simulink model "pneumatics"  (R2025a)
settings: Solver=FixedStepAuto  StartTime=0.0  StopTime=10  FixedStep=0.05  RelTol=1e-3
model workspace (MAT data in the model file):
  BP_MAX_SERVICE_REDUCTION = Simulink.Parameter
  BP_MAX_SERVICE_REDUCTION.Value = 25
  BP_MAX_SERVICE_REDUCTION.Complexity = 'real'
  BP_MAX_SERVICE_REDUCTION.Dimensions = [1 1]
  BP_MAX_SERVICE_REDUCTION.DataType = 'auto'
  BP_MAX_SERVICE_REDUCTION.DocUnits = 'psig'
  BP_NOMINAL_PRESSURE = Simulink.Parameter
  BP_NOMINAL_PRESSURE.Value = 90
  BP_NOMINAL_PRESSURE.Complexity = 'real'
  BP_NOMINAL_PRESSURE.Dimensions = [1 1]
  BP_NOMINAL_PRESSURE.DataType = 'auto'
  BP_NOMINAL_PRESSURE.DocUnits = 'psig'
  MAIN_RES_NOMINAL_PRESSURE = Simulink.Parameter
  MAIN_RES_NOMINAL_PRESSURE.Value = 164.69
  MAIN_RES_NOMINAL_PRESSURE.Complexity = 'real'
  MAIN_RES_NOMINAL_PRESSURE.Dimensions = [1 1]
  MAIN_RES_NOMINAL_PRESSURE.DataType = 'auto'
  MAIN_RES_NOMINAL_PRESSURE.DocUnits = 'psig'
  RESERVOIR_TEMPERATURE = Simulink.Parameter
  RESERVOIR_TEMPERATURE.Value = 75
  RESERVOIR_TEMPERATURE.Complexity = 'real'
  RESERVOIR_TEMPERATURE.Dimensions = [1 1]
  RESERVOIR_TEMPERATURE.DataType = 'auto'
  RESERVOIR_TEMPERATURE.DocUnits = '°F'
  RESERVOIR_VOLUME = Simulink.Parameter
  RESERVOIR_VOLUME.Value = 10
  RESERVOIR_VOLUME.Complexity = 'real'
  RESERVOIR_VOLUME.Dimensions = [1 1]
  RESERVOIR_VOLUME.DataType = 'auto'
  RESERVOIR_VOLUME.DocUnits = 'gal'
  TRANSDUCER_ADC_OUTPUT_RANGE = Simulink.Parameter
  TRANSDUCER_ADC_OUTPUT_RANGE.Value = 1019
  TRANSDUCER_ADC_OUTPUT_RANGE.Complexity = 'real'
  TRANSDUCER_ADC_OUTPUT_RANGE.Dimensions = [1 1]
  TRANSDUCER_ADC_OUTPUT_RANGE.DataType = 'auto'
  TRANSDUCER_ADC_OUTPUT_RANGE.DocUnits = 'bit'
  TRANSDUCER_OUTPUT_HIGH = Simulink.Parameter
  TRANSDUCER_OUTPUT_HIGH.Value = 4.5
  TRANSDUCER_OUTPUT_HIGH.Complexity = 'real'
  TRANSDUCER_OUTPUT_HIGH.Dimensions = [1 1]
  TRANSDUCER_OUTPUT_HIGH.DataType = 'auto'
  TRANSDUCER_OUTPUT_LOW = Simulink.Parameter
  TRANSDUCER_OUTPUT_LOW.Value = 0.5
  TRANSDUCER_OUTPUT_LOW.Complexity = 'real'
  TRANSDUCER_OUTPUT_LOW.Dimensions = [1 1]
  TRANSDUCER_OUTPUT_LOW.DataType = 'auto'
  TRANSDUCER_OUTPUT_RANGE = Simulink.Parameter
  TRANSDUCER_OUTPUT_RANGE.Value = 4
  TRANSDUCER_OUTPUT_RANGE.Complexity = 'real'
  TRANSDUCER_OUTPUT_RANGE.Dimensions = [1 1]
  TRANSDUCER_OUTPUT_RANGE.DataType = 'auto'
  TRANSDUCER_OUTPUT_RANGE.DocUnits = 'V'
  TRANSDUCER_PRESSURE_RANGE = Simulink.Parameter
  TRANSDUCER_PRESSURE_RANGE.Value = 150
  TRANSDUCER_PRESSURE_RANGE.Complexity = 'real'
  TRANSDUCER_PRESSURE_RANGE.Dimensions = [1 1]
  TRANSDUCER_PRESSURE_RANGE.DataType = 'auto'
  TRANSDUCER_PRESSURE_RANGE.DocUnits = 'psig'
undefined symbols (not defined in the file or in its folder): max_bc_pressure
settings Model: DataDictionary=pneumatics.sldd  ExtModeTrigDuration=100  Creator=adam  LastModifiedBy=adam
settings SolverCC: MaxConsecutiveMinStep=3
settings OptimizationCC: DefaultParameterBehavior=Inlined  InlineInvariantSignals=on  EnhancedBackFolding=on  PassReuseOutputArgsThreshold=0.0  OptimizeBlockOrder=speed  DifferentSizesBufferReuse=on  OptimizationCustomize=off
settings DebuggingCC: ParameterTunabilityLossMsg=error
settings HardwareCC: TargetBitPerLong=64.0  TargetBitPerPointer=64.0  TargetBitPerSizeT=64.0  TargetBitPerPtrDiffT=64.0  TargetLongLongMode=on  TargetIntDivRoundTo=Zero  TargetEndianess=LittleEndian  TargetWordSize=64.0  TargetHWDeviceType=MATLAB Host  ProdEqTarget=off
settings SFSimCC: MATLABDynamicMemAlloc=off
settings RTWCC: PackageGeneratedCodeAndArtifacts=on  RetainRTWFile=on  GPUComputeCapability=3.5
settings CodeAppCC: ForceParamTrailComments=on  MaxIdLength=95.0  OperatorAnnotations=on
settings SimscapeCC: SimscapeLogOpenViewer=on  SimscapeLogLimitData=off

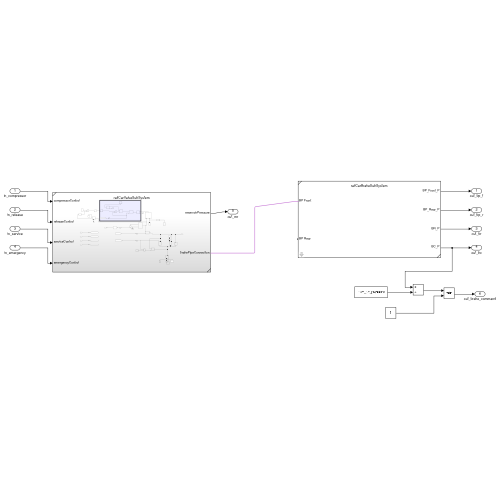
[thumbnail: Simulink's stored preview of the top-level diagram]
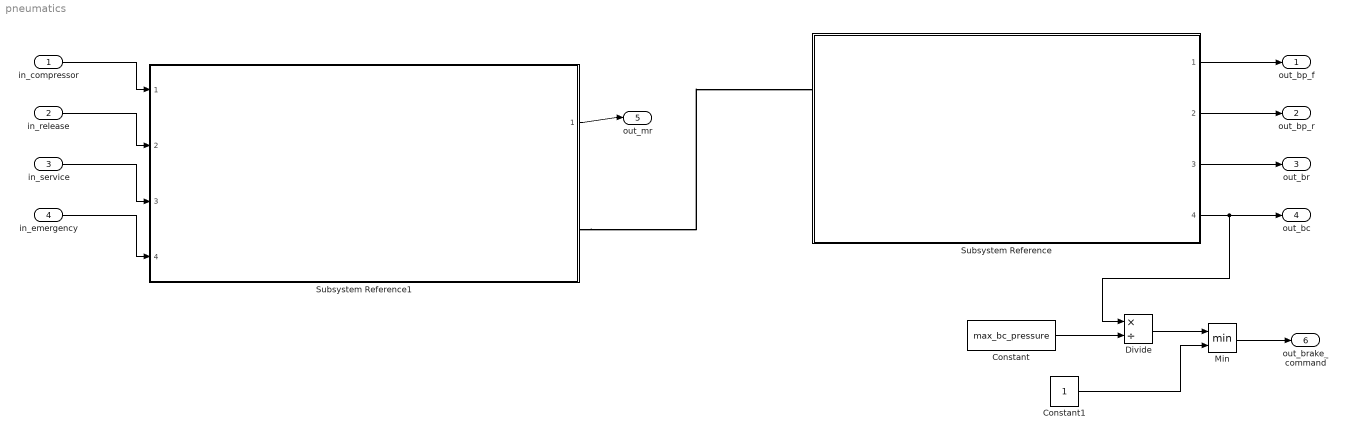
== system pneumatics ==
  in_compressor : Inport
  in_release : Inport  Port=2
  in_service : Inport  Port=3
  in_emergency : Inport  Port=4
  Constant : Constant  Value=max_bc_pressure
  Constant1 : Constant
  Divide : Product  Inputs=*/
  Min : MinMax  Inputs=2
  Subsystem Reference : Subsystem  ReferencedSubsystem=railCarBrakeSubSystem  reservoir_temperature=RESERVOIR_TEMPERATURE degF  p_init=BP_NOMINAL_PRESSURE psi  r_volume=10 gal  bc_volume=4 gal  bc_pressure=14.69 psi  length=50 ft  area=1.23 in^2  Dh=1.25 in
  Subsystem Reference1 : Subsystem  ReferencedSubsystem=railCarValveSubSystem
  out_bp_f : Outport
  out_bp_r : Outport  Port=2
  out_br : Outport  Port=3
  out_bc : Outport  Port=4
  out_mr : Outport  Port=5
  out_brake_command : Outport  Port=6
  wires:
  Subsystem Reference1/1 -> out_mr/1
  Subsystem Reference/1 -> out_bp_f/1
  Subsystem Reference/2 -> out_bp_r/1
  Subsystem Reference/3 -> out_br/1
  Subsystem Reference/4 -> Divide/1, out_bc/1
  in_compressor/1 -> Subsystem Reference1/1
  in_release/1 -> Subsystem Reference1/2
  in_service/1 -> Subsystem Reference1/3
  in_emergency/1 -> Subsystem Reference1/4
  Constant/1 -> Divide/2
  Min/1 -> out_brake_command/1
  Divide/1 -> Min/1
  Constant1/1 -> Min/2
  connections:
  Subsystem Reference1/RConn1 -- Subsystem Reference/LConn1
